simulink model "gyroscope"  (R2023b)
settings: Solver=VariableStepAuto  StartTime=0.0  StopTime=10.0  RelTol=1e-3
values from neighbouring files (symbols this model uses):
  BiasStability = BiasStability/3600    (= 4.62962962963e-08)    [Astrix200Specs.m]
  StdDevARW = ARW/Ts    (= 0.01)    [Astrix200Specs.m]
  Ts = 1/f    (= 0.01)    [Astrix200Specs.m]
undefined symbols (not defined in the file or in its folder): Ab, As, b, DiscIntNeverNeededParam, s
settings Model: Creator=matte  LastModifiedBy=matte

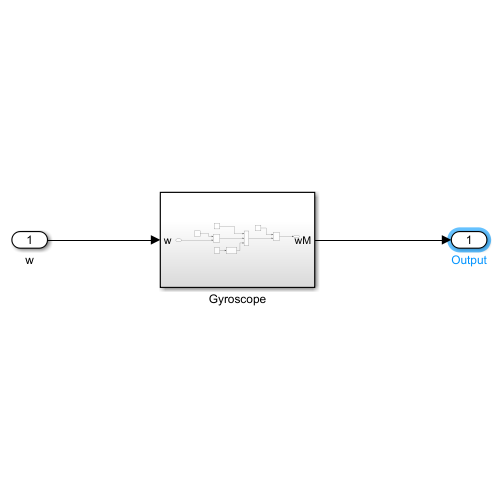
[thumbnail: Simulink's stored preview of the top-level diagram]
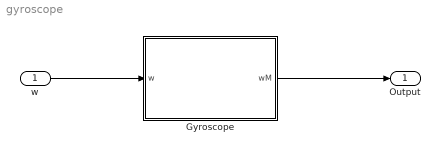
== system gyroscope ==
  w : Inport
  Gyroscope : Subsystem
  Output : Outport
  wires:
  w/1 -> Gyroscope/1(w)
  Gyroscope/1(wM) -> Output/1

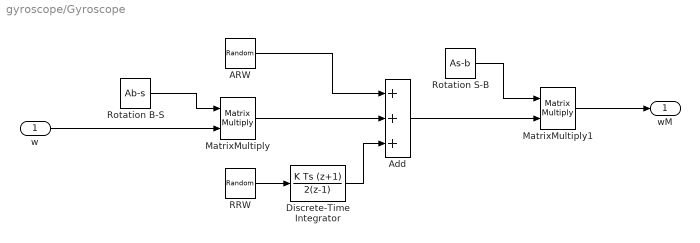
== system gyroscope/Gyroscope ==
  w : Inport
  ARW : RandomNumber  Variance=StdDevARW  Seed=12984537  SampleTime=Ts  VectorParams1D=off
  Add : Sum  Inputs=+++
  Discrete-Time Integrator : DiscreteIntegrator  IntegratorMethod=Integration: Trapezoidal  SampleTime=Ts  ICPrevOutput=DiscIntNeverNeededParam  ICPrevScaledInput=DiscIntNeverNeededParam
  MatrixMultiply : Product  Multiplication=Matrix(*)
  MatrixMultiply1 : Product  Multiplication=Matrix(*)
  RRW : RandomNumber  Variance=BiasStability  Seed=34654365  SampleTime=Ts  VectorParams1D=off
  Rotation B-S : Constant  Value=Ab-s
  Rotation S-B : Constant  Value=As-b
  wM : Outport
  wires:
  Add/1 -> MatrixMultiply1/2
  Rotation S-B/1 -> MatrixMultiply1/1
  Discrete-Time Integrator/1 -> Add/3
  MatrixMultiply/1 -> Add/2
  w/1 -> MatrixMultiply/2
  Rotation B-S/1 -> MatrixMultiply/1
  ARW/1 -> Add/1
  RRW/1 -> Discrete-Time Integrator/1
  MatrixMultiply1/1 -> wM/1
